simulink model "Angular_Input_Sliding_Mode_2"  (R2021b)
settings: Solver=VariableStepAuto  StartTime=0  StopTime=tspan(2)  RelTol=1e-8
undefined symbols (not defined in the file): Angle_max, BL_gain, K_switch, lambda_x_num, lambda_y_num, r_sim, tau_angle, Tmax, x_0
libraries: cstblocks x4
(part 1 of 2)
settings Model: Creator=domin  LastModifiedBy=domin
settings SolverCC: AlgebraicLoopSolver=TrustRegion
settings DataIOCC: SaveFormat=StructureWithTime
settings OptimizationCC: BlockReduction=off  BufferReuse=off
settings DebuggingCC: AlgebraicLoopMsg=none  UnconnectedInputMsg=none  UnconnectedOutputMsg=none  UnconnectedLineMsg=none  SFMachineParentedDataDiag=warning

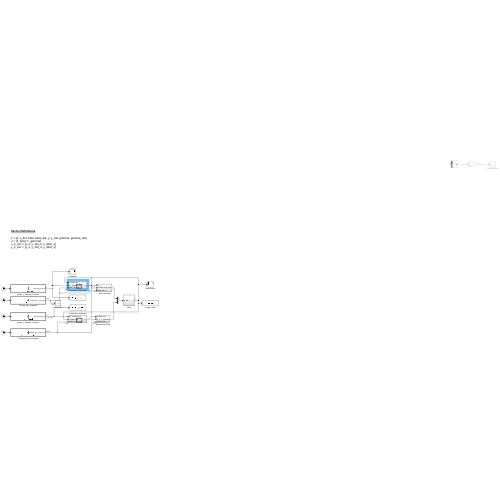
[thumbnail: Simulink's stored preview of the top-level diagram]
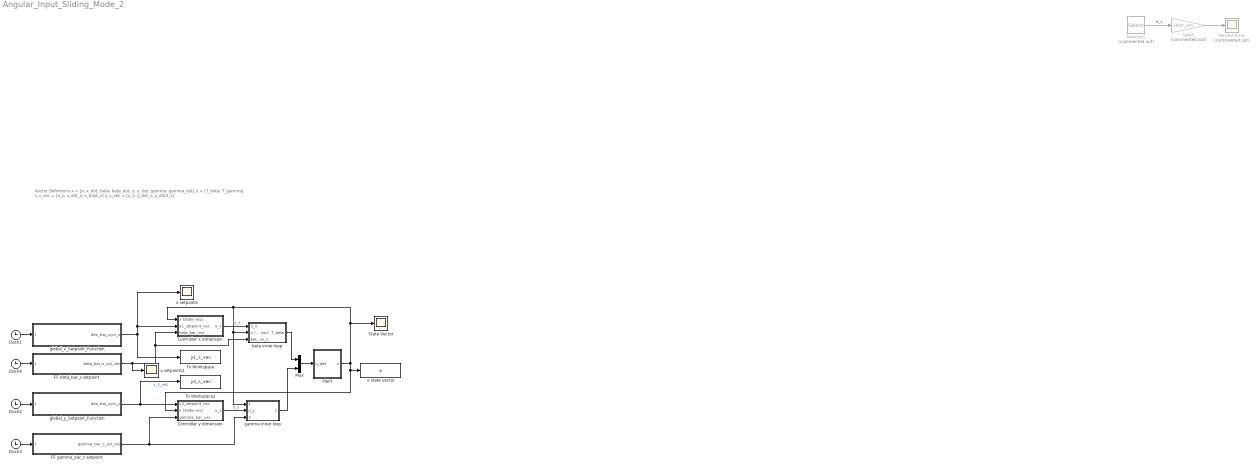
== system Angular_Input_Sliding_Mode_2 ==
  note: Vector Definitions
      |
      | x = [x; x_dot; beta; beta_dot; y; y_dot; gamma; gamma_dot]
      | u = [T_beta; T_gamma]
      | x_s_vec = [x_s; x_dot_s; x_ddot_s]
      | y_s_vec = [y_s; y_dot_s; y_ddot_s]
  Clock{1..4} (4 alike) : Clock
  Controller x dimension : Subsystem
  Controller y dimension : Subsystem
  FF beta_bar_s setpoint : MATLAB Function  TreatAsAtomicUnit=on
  FF gamma_bar_s setpoint : MATLAB Function  TreatAsAtomicUnit=on
  Gain5 : Gain  Commented=on  Gain=100/r_sim
  Mux : Mux  Inputs=2
  Percent Error : Scope  Commented=on
  Plant : Subsystem
  Selector1 : Selector  Commented=on  InputPortWidth=5  IndexOptions=Index vector (dialog)  Indices=[1]  OutputSizes=1
  State Vector : Scope
  To Workspace : ToWorkspace  VariableName=y1_s_vec  SampleTime=-1
  To Workspace2 : ToWorkspace  VariableName=y2_s_vec  SampleTime=-1
  beta inner loop : Subsystem
  gamma inner loop : Subsystem
  global_x_Setpoint_Function : MATLAB Function  TreatAsAtomicUnit=on
  global_y_Setpoint_Function : MATLAB Function  TreatAsAtomicUnit=on
  x setpoints : Scope
  x setpoints1 : Scope
  x state vector : ToWorkspace  VariableName=x  SampleTime=-1
  wires:
  Clock1/1 -> global_x_Setpoint_Function/1(t)
  Gain5/1 -> Percent Error/1
  Selector1/1 -> Gain5/1  "e_x"
  Clock2/1 -> global_y_Setpoint_Function/1(t)
  Controller x dimension/1(u_x) -> beta inner loop/1(u_x)  "u_x"
  Controller y dimension/1(u_y) -> gamma inner loop/2(u_y)  "u_y"
  global_x_Setpoint_Function/1(des_traj_sym_x) -> x setpoints/1, Controller x dimension/2(y1_setpoint_vec), To Workspace/1
  global_y_Setpoint_Function/1(des_traj_sym_y) -> To Workspace2/1, Controller y dimension/1(y2_setpoint_vec)  "y_s_vec"
  Plant/1(x) -> x state vector/1, Controller y dimension/2(x (state vec)), gamma inner loop/1(x (state vec)), beta inner loop/2(x (state vec)), Controller x dimension/1(x (state vec)), State Vector/1
  beta inner loop/1(T_beta) -> Mux/1
  Mux/1 -> Plant/1(u_des)
  gamma inner loop/1(T_gamma) -> Mux/2
  Clock3/1 -> FF gamma_bar_s setpoint/1(t)
  Clock4/1 -> FF beta_bar_s setpoint/1(t)
  FF beta_bar_s setpoint/1(beta_bar_s_sol_vec) -> x setpoints1/1, Controller x dimension/3(beta_bar_vec), beta inner loop/3(beta_bar_s)
  FF gamma_bar_s setpoint/1(gamma_bar_s_sol_vec) -> gamma inner loop/3(gamma_bar_s), Controller y dimension/3(gamma_bar_vec)

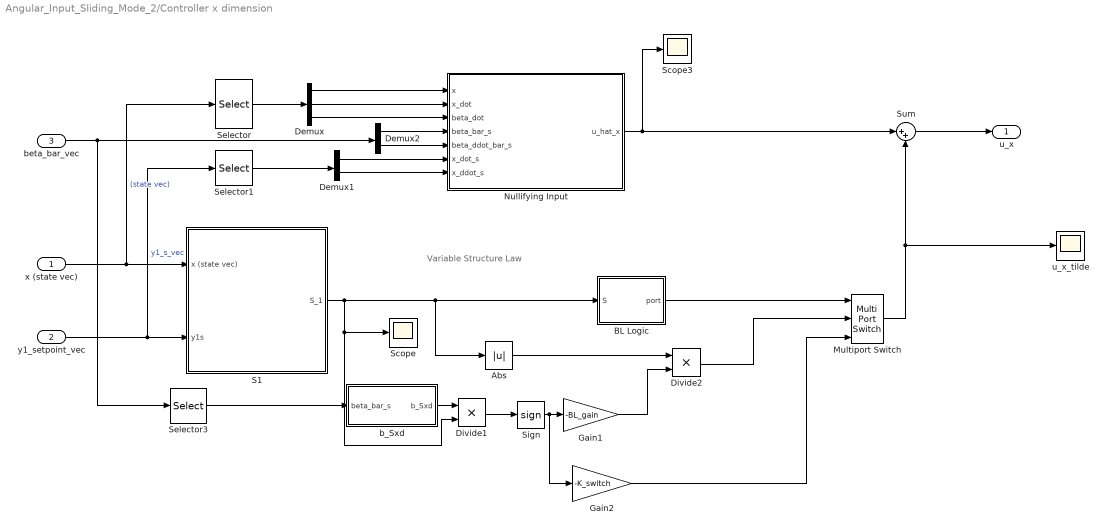
== system Angular_Input_Sliding_Mode_2/Controller x dimension ==
  note: Variable Structure Law
  x (state vec) : Inport
  y1_setpoint_vec : Inport  Port=2
  beta_bar_vec : Inport  Port=3
  Abs : Abs
  BL Logic : MATLAB Function  TreatAsAtomicUnit=on
  Demux : Demux  Outputs=3
  Demux1 : Demux  Outputs=2
  Demux2 : Demux  Outputs=2
  Divide1 : Product  Inputs=**
  Divide2 : Product  Inputs=**
  Gain1 : Gain  Gain=-BL_gain
  Gain2 : Gain  Gain=-K_switch
  Multiport Switch : MultiPortSwitch  Inputs=2
  Nullifying Input : MATLAB Function  TreatAsAtomicUnit=on
  S1 : Subsystem
  Scope : Scope
  Scope3 : Scope
  Selector : Selector  InputPortWidth=8  IndexOptions=Index vector (dialog)  Indices=[1 2 4]  OutputSizes=1
  Selector1 : Selector  InputPortWidth=3  IndexOptions=Index vector (dialog)  Indices=[2 3]  OutputSizes=1
  Selector3 : Selector  InputPortWidth=2  IndexOptions=Index vector (dialog)  Indices=[1]  OutputSizes=1
  Sign : Signum
  Sum : Sum  Inputs=|++
  b_Sxd : MATLAB Function  TreatAsAtomicUnit=on
  u_x_tilde : Scope
  u_x : Outport
  wires:
  Sum/1 -> u_x/1
  x (state vec)/1 -> S1/1(x (state vec)), Selector/1  "(state vec)"
  y1_setpoint_vec/1 -> Selector1/1, S1/2(y1s)  "y1_s_vec"
  Selector/1 -> Demux/1
  Demux/2 -> Nullifying Input/2(x_dot)
  Selector1/1 -> Demux1/1
  Demux1/1 -> Nullifying Input/6(x_dot_s)
  Demux1/2 -> Nullifying Input/7(x_ddot_s)
  Nullifying Input/1(u_hat_x) -> Scope3/1, Sum/1
  b_Sxd/1(b_Sxd) -> Divide1/1
  Divide2/1 -> Multiport Switch/2
  S1/1(S_1) -> Divide1/2, Scope/1, Abs/1, BL Logic/1(S)
  Demux/1 -> Nullifying Input/1(x)
  Gain1/1 -> Divide2/2
  BL Logic/1(port) -> Multiport Switch/1
  Multiport Switch/1 -> Sum/2, u_x_tilde/1
  Sign/1 -> Gain2/1, Gain1/1
  Divide1/1 -> Sign/1
  Gain2/1 -> Multiport Switch/3
  Abs/1 -> Divide2/1
  Demux/3 -> Nullifying Input/3(beta_dot)
  Demux2/1 -> Nullifying Input/4(beta_bar_s)
  Demux2/2 -> Nullifying Input/5(beta_ddot_bar_s)
  beta_bar_vec/1 -> Demux2/1, Selector3/1
  Selector3/1 -> b_Sxd/1(beta_bar_s)

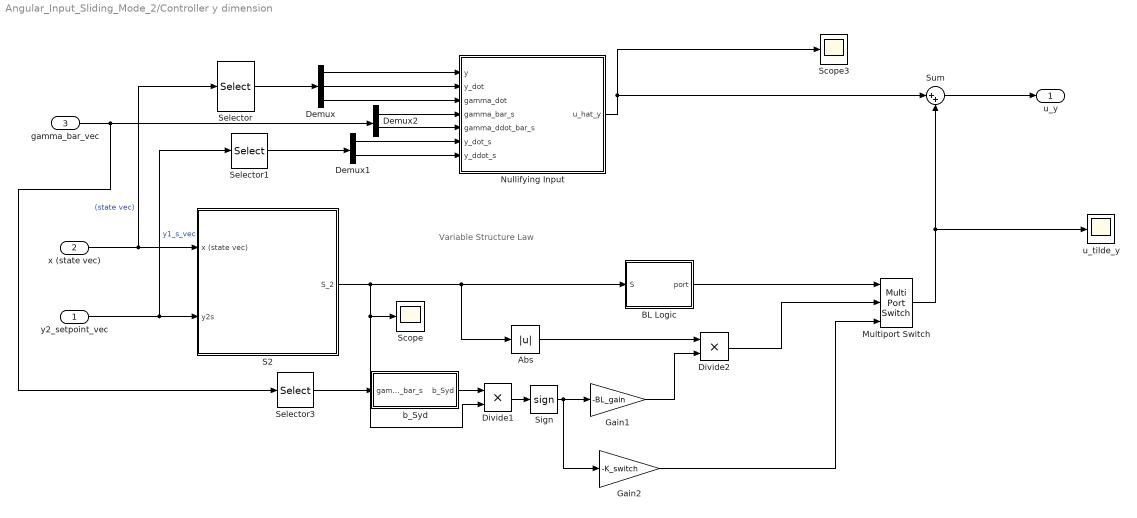
== system Angular_Input_Sliding_Mode_2/Controller y dimension ==
  note: Variable Structure Law
  y2_setpoint_vec : Inport
  x (state vec) : Inport  Port=2
  gamma_bar_vec : Inport  Port=3
  Abs : Abs
  BL Logic : MATLAB Function  TreatAsAtomicUnit=on
  Demux : Demux  Outputs=3
  Demux1 : Demux  Outputs=2
  Demux2 : Demux  Outputs=2
  Divide1 : Product  Inputs=**
  Divide2 : Product  Inputs=**
  Gain1 : Gain  Gain=-BL_gain
  Gain2 : Gain  Gain=-K_switch
  Multiport Switch : MultiPortSwitch  Inputs=2
  Nullifying Input : MATLAB Function  TreatAsAtomicUnit=on
  S2 : Subsystem
  Scope : Scope
  Scope3 : Scope
  Selector : Selector  InputPortWidth=8  IndexOptions=Index vector (dialog)  Indices=[5 6 8]  OutputSizes=1
  Selector1 : Selector  InputPortWidth=3  IndexOptions=Index vector (dialog)  Indices=[2 3]  OutputSizes=1
  Selector3 : Selector  InputPortWidth=2  IndexOptions=Index vector (dialog)  Indices=[1]  OutputSizes=1
  Sign : Signum
  Sum : Sum  Inputs=|++
  b_Syd : MATLAB Function  TreatAsAtomicUnit=on
  u_tilde_y : Scope
  u_y : Outport
  wires:
  Sum/1 -> u_y/1
  Gain1/1 -> Divide2/2
  Abs/1 -> Divide2/1
  Gain2/1 -> Multiport Switch/3
  Multiport Switch/1 -> Sum/2, u_tilde_y/1
  BL Logic/1(port) -> Multiport Switch/1
  Sign/1 -> Gain1/1, Gain2/1
  b_Syd/1(b_Syd) -> Divide1/1
  Divide2/1 -> Multiport Switch/2
  S2/1(S_2) -> Abs/1, BL Logic/1(S), Divide1/2, Scope/1
  Divide1/1 -> Sign/1
  Demux/3 -> Nullifying Input/3(gamma_dot)
  Demux/1 -> Nullifying Input/1(y)
  Nullifying Input/1(u_hat_y) -> Scope3/1, Sum/1
  Selector/1 -> Demux/1
  Demux/2 -> Nullifying Input/2(y_dot)
  x (state vec)/1 -> Selector/1, S2/1(x (state vec))  "(state vec)"
  y2_setpoint_vec/1 -> Selector1/1, S2/2(y2s)  "y1_s_vec"
  Demux1/2 -> Nullifying Input/7(y_ddot_s)
  Demux1/1 -> Nullifying Input/6(y_dot_s)
  Selector1/1 -> Demux1/1
  Selector3/1 -> b_Syd/1(gamma_bar_s)
  Demux2/1 -> Nullifying Input/4(gamma_bar_s)
  Demux2/2 -> Nullifying Input/5(gamma_ddot_bar_s)
  gamma_bar_vec/1 -> Demux2/1, Selector3/1

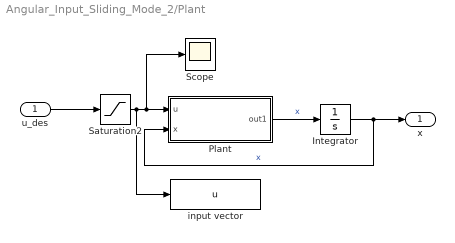
== system Angular_Input_Sliding_Mode_2/Plant ==
  u_des : Inport
  Integrator : Integrator  InitialCondition=x_0
  Plant : Subsystem
  Saturation2 : Saturate  UpperLimit=Tmax  LowerLimit=-Tmax  ZeroCross=off
  Scope : Scope
  input vector : ToWorkspace  VariableName=u  SampleTime=-1
  x : Outport
  wires:
  Saturation2/1 -> Scope/1, Plant/1(u), input vector/1
  Integrator/1 -> x/1, Plant/2(x)  "x"
  Plant/1(out1) -> Integrator/1  "x"
  u_des/1 -> Saturation2/1

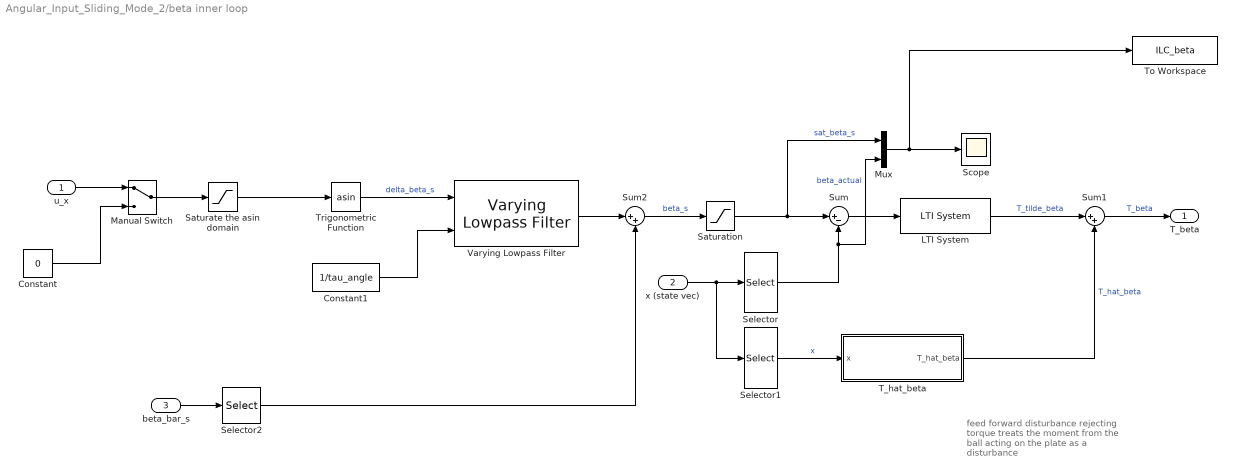
== system Angular_Input_Sliding_Mode_2/beta inner loop ==
  note: feed forward disturbance rejecting torque treats the moment from the ball acting on the plate as a disturbance
  u_x : Inport
  x (state vec) : Inport  Port=2
  beta_bar_s : Inport  Port=3
  Constant : Constant  Value=0
  Constant1 : Constant  Value=1/tau_angle
  LTI System : cstblocks/LTI System  sys=C_beta  IC=[]
  Manual Switch : ManualSwitch
  Mux : Mux  Inputs=2
  Saturate the asin domain : Saturate  UpperLimit=1  LowerLimit=-1
  Saturation : Saturate  UpperLimit=Angle_max  LowerLimit=-Angle_max
  Scope : Scope
  Selector : Selector  InputPortWidth=8  IndexOptions=Index vector (dialog)  Indices=[3]  OutputSizes=1
  Selector1 : Selector  InputPortWidth=8  IndexOptions=Index vector (dialog)  Indices=[1]  OutputSizes=1
  Selector2 : Selector  InputPortWidth=2  IndexOptions=Index vector (dialog)  Indices=[1 ]  OutputSizes=1
  Sum : Sum  Inputs=|+-
  Sum1 : Sum  Inputs=|++
  Sum2 : Sum  Inputs=|++
  T_hat_beta : MATLAB Function  TreatAsAtomicUnit=on
  To Workspace : ToWorkspace  VariableName=ILC_beta  SampleTime=-1
  Trigonometric Function : Trigonometry  Operator=asin
  Varying Lowpass Filter : cstblocks/Linear Parameter Varying/Varying Lowpass Filter  N=1
  T_beta : Outport
  wires:
  u_x/1 -> Manual Switch/1
  Trigonometric Function/1 -> Varying Lowpass Filter/1  "delta_beta_s"
  x (state vec)/1 -> Selector1/1, Selector/1
  Selector/1 -> Mux/2, Sum/2  "beta_actual"
  Sum/1 -> LTI System/1
  Saturate the asin domain/1 -> Trigonometric Function/1
  LTI System/1 -> Sum1/1  "T_tilde_beta"
  T_hat_beta/1(T_hat_beta) -> Sum1/2  "T_hat_beta"
  Sum1/1 -> T_beta/1  "T_beta"
  Selector1/1 -> T_hat_beta/1(x)  "x"
  Constant/1 -> Manual Switch/2
  Manual Switch/1 -> Saturate the asin domain/1
  Constant1/1 -> Varying Lowpass Filter/2
  Varying Lowpass Filter/1 -> Sum2/1
  Mux/1 -> To Workspace/1, Scope/1
  Saturation/1 -> Mux/1, Sum/1  "sat_beta_s"
  beta_bar_s/1 -> Selector2/1
  Selector2/1 -> Sum2/2
  Sum2/1 -> Saturation/1  "beta_s"

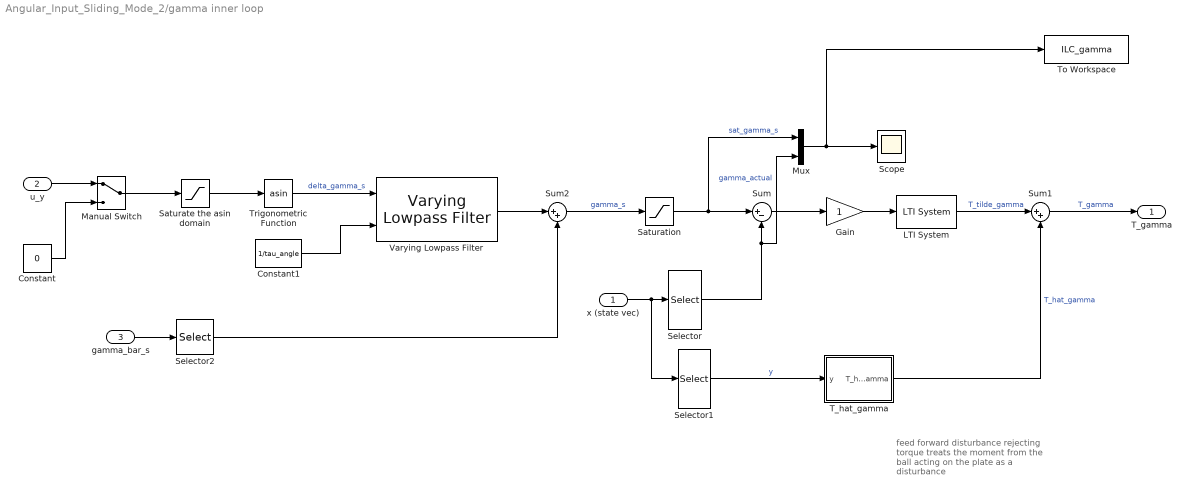
== system Angular_Input_Sliding_Mode_2/gamma inner loop ==
  note: feed forward disturbance rejecting torque treats the moment from the ball acting on the plate as a disturbance
  x (state vec) : Inport
  u_y : Inport  Port=2
  gamma_bar_s : Inport  Port=3
  Constant : Constant  Value=0
  Constant1 : Constant  Value=1/tau_angle
  Gain : Gain
  LTI System : cstblocks/LTI System  sys=C_gamma  IC=[]
  Manual Switch : ManualSwitch
  Mux : Mux  Inputs=2
  Saturate the asin domain : Saturate  UpperLimit=1  LowerLimit=-1
  Saturation : Saturate  UpperLimit=Angle_max  LowerLimit=-Angle_max
  Scope : Scope
  Selector : Selector  InputPortWidth=8  IndexOptions=Index vector (dialog)  Indices=[7]  OutputSizes=1
  Selector1 : Selector  InputPortWidth=8  IndexOptions=Index vector (dialog)  Indices=[5]  OutputSizes=1
  Selector2 : Selector  InputPortWidth=2  IndexOptions=Index vector (dialog)  Indices=[1 ]  OutputSizes=1
  Sum : Sum  Inputs=|+-
  Sum1 : Sum  Inputs=|++
  Sum2 : Sum  Inputs=|++
  T_hat_gamma : MATLAB Function  TreatAsAtomicUnit=on
  To Workspace : ToWorkspace  VariableName=ILC_gamma  SampleTime=-1
  Trigonometric Function : Trigonometry  Operator=asin
  Varying Lowpass Filter : cstblocks/Linear Parameter Varying/Varying Lowpass Filter  N=1
  T_gamma : Outport
  wires:
  LTI System/1 -> Sum1/1  "T_tilde_gamma"
  Sum/1 -> Gain/1
  Selector/1 -> Mux/2, Sum/2  "gamma_actual"
  Trigonometric Function/1 -> Varying Lowpass Filter/1  "delta_gamma_s"
  Saturation/1 -> Mux/1, Sum/1  "sat_gamma_s"
  Saturate the asin domain/1 -> Trigonometric Function/1
  T_hat_gamma/1(T_hat_gamma) -> Sum1/2  "T_hat_gamma"
  x (state vec)/1 -> Selector1/1, Selector/1
  Selector1/1 -> T_hat_gamma/1(y)  "y"
  Sum1/1 -> T_gamma/1  "T_gamma"
  u_y/1 -> Manual Switch/1
  Constant/1 -> Manual Switch/2
  Manual Switch/1 -> Saturate the asin domain/1
  Gain/1 -> LTI System/1
  Constant1/1 -> Varying Lowpass Filter/2
  Varying Lowpass Filter/1 -> Sum2/1
  Mux/1 -> To Workspace/1, Scope/1
  gamma_bar_s/1 -> Selector2/1
  Sum2/1 -> Saturation/1  "gamma_s"
  Selector2/1 -> Sum2/2

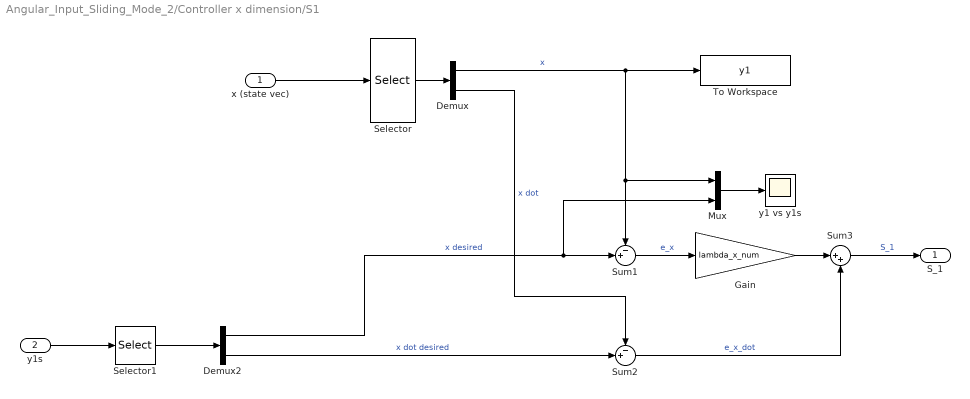
== system Angular_Input_Sliding_Mode_2/Controller x dimension/S1 ==
  x (state vec) : Inport
  y1s : Inport  Port=2
  Demux : Demux  Outputs=2
  Demux2 : Demux  Outputs=2
  Gain : Gain  Gain=lambda_x_num
  Mux : Mux  Inputs=2
  Selector : Selector  InputPortWidth=8  IndexOptions=Index vector (dialog)  Indices=[1 2]  OutputSizes=1
  Selector1 : Selector  InputPortWidth=3  IndexOptions=Index vector (dialog)  Indices=[1 2]  OutputSizes=1
  Sum1 : Sum  Inputs=-+|
  Sum2 : Sum  Inputs=-+|
  Sum3 : Sum  Inputs=|++
  To Workspace : ToWorkspace  VariableName=y1  SampleTime=-1
  y1 vs y1s : Scope
  S_1 : Outport
  wires:
  Demux/1 -> Sum1/1, Mux/1, To Workspace/1  "x"
  Demux2/2 -> Sum2/2  "x dot desired"
  Sum3/1 -> S_1/1  "S_1"
  y1s/1 -> Selector1/1
  Mux/1 -> y1 vs y1s/1
  Selector1/1 -> Demux2/1
  Selector/1 -> Demux/1
  Sum2/1 -> Sum3/2  "e_x_dot"
  Demux/2 -> Sum2/1  "x dot"
  x (state vec)/1 -> Selector/1
  Demux2/1 -> Mux/2, Sum1/2  "x desired"
  Gain/1 -> Sum3/1
  Sum1/1 -> Gain/1  "e_x"

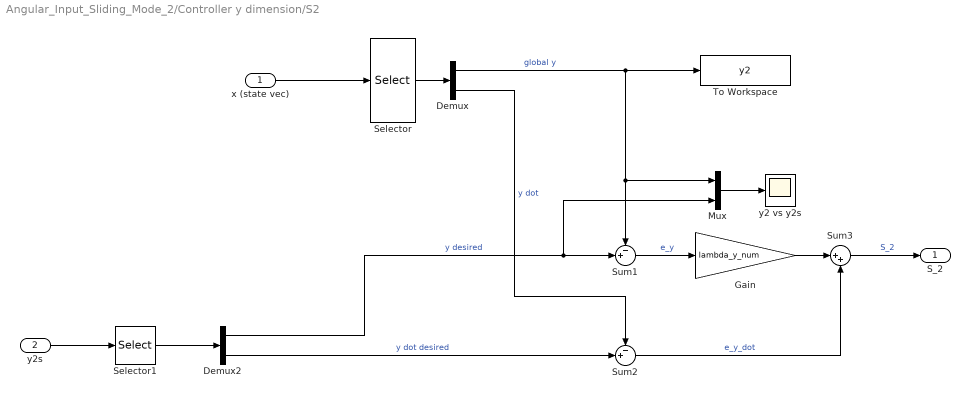
== system Angular_Input_Sliding_Mode_2/Controller y dimension/S2 ==
  x (state vec) : Inport
  y2s : Inport  Port=2
  Demux : Demux  Outputs=2
  Demux2 : Demux  Outputs=2
  Gain : Gain  Gain=lambda_y_num
  Mux : Mux  Inputs=2
  Selector : Selector  InputPortWidth=8  IndexOptions=Index vector (dialog)  Indices=[5 6]  OutputSizes=1
  Selector1 : Selector  InputPortWidth=3  IndexOptions=Index vector (dialog)  Indices=[1 2]  OutputSizes=1
  Sum1 : Sum  Inputs=-+|
  Sum2 : Sum  Inputs=-+|
  Sum3 : Sum  Inputs=|++
  To Workspace : ToWorkspace  VariableName=y2  SampleTime=-1
  y2 vs y2s : Scope
  S_2 : Outport
  wires:
  Sum3/1 -> S_2/1  "S_2"
  Sum1/1 -> Gain/1  "e_y"
  Sum2/1 -> Sum3/2  "e_y_dot"
  x (state vec)/1 -> Selector/1
  Gain/1 -> Sum3/1
  Demux/1 -> Sum1/1, Mux/1, To Workspace/1  "global y"
  Demux2/1 -> Mux/2, Sum1/2  "y desired"
  Demux2/2 -> Sum2/2  "y dot desired"
  y2s/1 -> Selector1/1
  Demux/2 -> Sum2/1  "y dot"
  Selector1/1 -> Demux2/1
  Mux/1 -> y2 vs y2s/1
  Selector/1 -> Demux/1

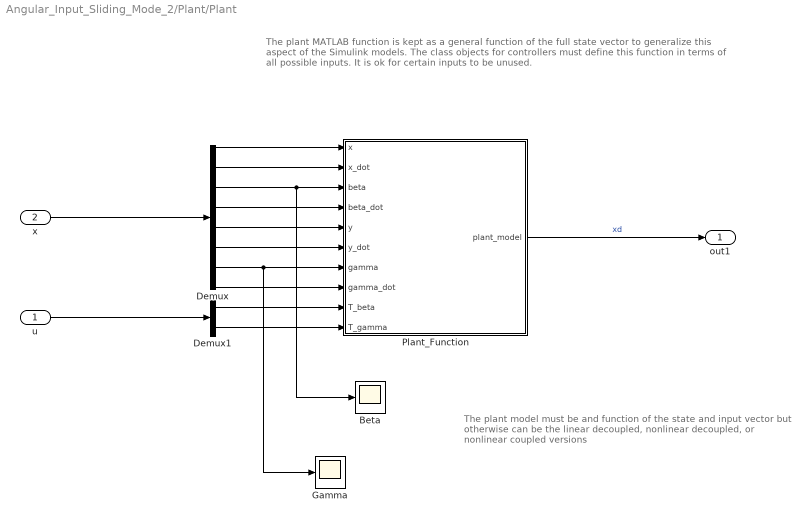
== system Angular_Input_Sliding_Mode_2/Plant/Plant ==
  note: The plant MATLAB function is kept as a general function of the full state vector
      | to generalize this aspect of the Simulink models. The class objects for controllers must define this function in terms of all possible inputs. It is ok for certain inputs to be unused.
  note: The plant model must be and function of the state and input vector
      |  but otherwise can be the linear decoupled, nonlinear decoupled,
      | or nonlinear coupled versions
  u : Inport
  x : Inport  Port=2
  Beta : Scope
  Demux : Demux  Outputs=8
  Demux1 : Demux  Outputs=2
  Gamma : Scope
  Plant_Function : MATLAB Function  TreatAsAtomicUnit=on
  out1 : Outport
  wires:
  Demux1/1 -> Plant_Function/9(T_beta)
  Demux1/2 -> Plant_Function/10(T_gamma)
  Demux/5 -> Plant_Function/5(y)
  Demux/8 -> Plant_Function/8(gamma_dot)
  Demux/1 -> Plant_Function/1(x)
  Demux/3 -> Beta/1, Plant_Function/3(beta)
  Demux/4 -> Plant_Function/4(beta_dot)
  Demux/2 -> Plant_Function/2(x_dot)
  Demux/6 -> Plant_Function/6(y_dot)
  x/1 -> Demux/1
  Plant_Function/1(plant_model) -> out1/1  "xd"
  u/1 -> Demux1/1
  Demux/7 -> Gamma/1, Plant_Function/7(gamma)

== matlab function Angular_Input_Sliding_Mode_2/FF gamma_bar_s setpoint ==
  data: t input; gamma_bar_s_sol_vec output
function gamma_bar_s_sol_vec = gamma_bar_s_vec(t)
%#codegen

%    This function was generated by the Symbolic Math Toolbox version 9.0.
%    22-Feb-2022 16:55:39

t2 = t.*pi;
t3 = pi.^2;
t4 = pi.^3;
t7 = t./2.0;
t21 = 5.151844329946315e+2;
t5 = cos(t2);
t6 = sin(t2);
t8 = t2./3.0;
t11 = -t7;
t14 = t3./9.0;
t26 = t3+6.294917864476386e+1;
t32 = t21.*(1.5e+1./9.74e+2);
t34 = t.*t21.*(-1.5e+1./9.74e+2);
t43 = t21.*3.286251181360353e-7;
t9 = t5.*pi;
t10 = t6.*pi;
t12 = cos(t8);
t13 = sin(t8);
t17 = t3.*t5;
t18 = t4.*t5;
t19 = t3.*t6;
t20 = t4.*t6;
t31 = 1.0./t26;
t33 = t.*t32;
t35 = t14+6.294917864476386e+1;
t37 = exp(t34);
t38 = t32+1.0./2.0;
t39 = t6.*t32;
t40 = t32-1.0./2.0;
t41 = t6.*t21.*(-1.5e+1./9.74e+2);
t57 = t11+t34;
t92 = t43+2.686510340762089e-3;
t96 = t43-2.686510340762089e-3;
t15 = -t9;
t16 = -t10;
t22 = (t12.*pi)./3.0;
t23 = (t13.*pi)./3.0;
t27 = t12.*t14;
t28 = (t4.*t12)./2.7e+1;
t29 = t13.*t14;
t30 = (t4.*t13)./2.7e+1;
t36 = exp(t33);
t42 = t9.*t32;
t44 = 1.0./t35;
t45 = t38.^2;
t46 = t9.*t21.*(-1.5e+1./9.74e+2);
t47 = t19.*t32;
t48 = t13.*t32;
t49 = t40.^2;
t50 = t12.*t21.*pi.*(5.0./9.74e+2);
t51 = t13.*t21.*(-1.5e+1./9.74e+2);
t52 = t11+t33;
t54 = t5.*t38;
t55 = t3.*t13.*t21.*1.711156741957563e-3;
t56 = t6.*t38;
t59 = t5.*t40;
t60 = t6.*t40;
t61 = t9.*t38;
t62 = t10.*t38;
t64 = exp(t57);
t65 = t9.*t40;
t66 = t10.*t40;
t68 = t9+t39;
t69 = t12.*t38;
t70 = t13.*t38;
t72 = t19.*t38;
t73 = t9+t41;
t74 = t12.*t40;
t75 = t13.*t40;
t77 = t19.*t40;
t24 = -t22;
t25 = -t23;
t53 = -t50;
t58 = exp(t52);
t63 = t3+t45;
t67 = t3+t49;
t71 = t15.*t38;
t76 = t16.*t40;
t79 = t19+t42;
t81 = t19+t46;
t82 = -t77;
t83 = t14+t45;
t84 = t22.*t38;
t85 = t23.*t38;
t86 = t9+t56;
t87 = t14+t49;
t88 = t22.*t40;
t89 = t69.*pi.*(-1.0./3.0);
t90 = t23.*t40;
t91 = t10+t59;
t94 = t75.*pi.*(-1.0./3.0);
t95 = t16+t54;
t98 = t17+t62;
t99 = t15+t60;
t100 = t29.*t38;
t101 = t19+t65;
t102 = t29.*t40;
t103 = t22+t48;
t105 = t18+t72;
t106 = t3.*t75.*(-1.0./9.0);
t107 = t22+t51;
t109 = t29+t50;
t112 = t22+t70;
t113 = t23+t74;
t123 = t64.*t96;
t124 = t3.*t21.*t31.*t37.*t68.*1.648361999133433e-4;
t125 = t3.*t21.*t31.*t36.*t73.*1.648361999133433e-4;
t78 = 1.0./t63;
t80 = 1.0./t67;
t93 = 1.0./t83;
t97 = 1.0./t87;
t104 = t19+t71;
t108 = t17+t76;
t110 = t29+t53;
t111 = t18+t82;
t114 = t25+t69;
t115 = t24+t75;
t116 = t27+t85;
t117 = t29+t88;
t118 = t29+t89;
t119 = t27+t94;
t120 = t28+t100;
t121 = t28+t106;
t122 = t58.*t92;
t126 = -t124;
t127 = -t125;
t128 = t3.*t21.*t37.*t44.*t103.*1.831513332370481e-5;
t129 = t3.*t21.*t36.*t44.*t107.*1.831513332370481e-5;
t130 = t21.*t64.*t78.*t86.*4.120904997833581e-5;
t132 = t21.*t58.*t80.*t91.*pi.*1.648361999133433e-4;
t134 = t21.*t64.*t78.*pi.*(t10-t54).*(-1.648361999133433e-4);
t135 = t3.*t21.*t64.*t78.*t86.*1.648361999133433e-4;
t136 = t21.*t58.*t80.*(t9-t60).*(-4.120904997833581e-5);
t137 = t3.*t21.*t58.*t80.*(t9-t60).*(-1.648361999133433e-4);
t138 = t3.*t21.*t58.*t80.*(t9-t60).*1.648361999133433e-4;
t139 = t21.*t64.*t93.*t112.*4.120904997833581e-5;
t140 = t21.*t58.*t97.*(t22-t75).*(-4.120904997833581e-5);
t141 = t21.*t64.*t93.*pi.*(t23-t69).*(-5.494539997111442e-5);
t142 = t21.*t58.*t97.*t113.*pi.*5.494539997111442e-5;
t143 = t3.*t21.*t64.*t93.*t112.*1.831513332370481e-5;
t144 = t21.*t58.*t97.*(t22-t75).*4.120904997833581e-5;
t145 = t21.*t64.*t93.*pi.*(t23-t69).*5.494539997111442e-5;
t147 = t3.*t21.*t58.*t97.*(t22-t75).*(-1.831513332370481e-5);
t131 = -t130;
t133 = -t132;
t146 = -t143;
t148 = t123+t126+t128+t131+t134+t135+t139+t145+t146;
t149 = t122+t127+t129+t133+t136+t138+t142+t144+t147;
et1 = t45.*t123+t45.*t134+t45.*t135+t45.*t139+t45.*t145-t3.*t31.*t37.*t81.*1.347535934291581+t3.*t37.*t44.*t110.*1.497262149212868e-1+t21.*t64.*t78.*t105.*4.120904997833581e-5-t21.*t64.*t93.*t120.*4.120904997833581e-5+t21.*t64.*t78.*pi.*(t20-t17.*t38).*1.648361999133433e-4-t21.*t64.*t93.*pi.*(t30-(t3.*t69)./9.0).*5.494539997111442e-5+t3.*t21.*t31.*t37.*(t18+t47).*1.648361999133433e-4-t3.*t21.*t37.*t44.*(t28+t55).*1.831513332370481e-5-t3.*t21.*t31.*t37.*t68.*1.037630339546905e-2+t3.*t21.*t37.*t44.*t103.*1.152922599496562e-3;
et2 = t3.*t21.*t64.*t78.*t105.*(-1.648361999133433e-4)-t21.*t45.*t64.*t78.*t86.*4.120904997833581e-5+t3.*t21.*t64.*t93.*t120.*1.831513332370481e-5-t21.*t38.*t64.*t78.*t104.*8.241809995667163e-5+t21.*t38.*t64.*t93.*t118.*8.241809995667163e-5+t3.*t21.*t38.*t64.*t78.*t104.*3.296723998266865e-4-t3.*t21.*t38.*t64.*t93.*t118.*3.663026664740961e-5-t3.*t21.*t45.*t64.*t93.*t112.*1.831513332370481e-5+t21.*t38.*t64.*t78.*t98.*pi.*3.296723998266865e-4-t21.*t38.*t64.*t93.*t116.*pi.*1.098907999422288e-4;
et3 = t49.*t122+t49.*t136+t49.*t138+t49.*t142+t49.*t144+t49.*t147+t3.*t31.*t36.*t79.*1.347535934291581-t3.*t36.*t44.*t109.*1.497262149212868e-1+t21.*t58.*t80.*t111.*4.120904997833581e-5-t21.*t58.*t97.*t121.*4.120904997833581e-5+t21.*t58.*t80.*pi.*(t20+t17.*t40).*1.648361999133433e-4-t21.*t58.*t97.*pi.*(t30+t27.*t40).*5.494539997111442e-5+t3.*t21.*t31.*t36.*(t18-t19.*t21.*(1.5e+1./9.74e+2)).*1.648361999133433e-4-t3.*t21.*t31.*t36.*t73.*1.037630339546905e-2+t3.*t21.*t36.*t44.*t107.*1.152922599496562e-3-t3.*t21.*t58.*t80.*t111.*1.648361999133433e-4;
et4 = t3.*t21.*t58.*t97.*t121.*1.831513332370481e-5+t21.*t40.*t58.*t80.*t101.*8.241809995667163e-5-t21.*t40.*t58.*t97.*t117.*8.241809995667163e-5-t3.*t21.*t36.*t44.*(t28-t55).*1.831513332370481e-5-t3.*t21.*t40.*t58.*t80.*t101.*3.296723998266865e-4+t3.*t21.*t40.*t58.*t97.*t117.*3.663026664740961e-5-t21.*t49.*t58.*t80.*t91.*pi.*1.648361999133433e-4-t21.*t40.*t58.*t80.*t108.*pi.*3.296723998266865e-4+t21.*t40.*t58.*t97.*t119.*pi.*1.098907999422288e-4;
et5 = t38.*t123+t38.*t134+t38.*t135+t38.*t139+t38.*t145-t3.*t31.*t37.*t68.*6.737679671457906e-1+t3.*t37.*t44.*t103.*7.486310746064339e-2-t21.*t64.*t78.*t104.*4.120904997833581e-5+t21.*t64.*t93.*t118.*4.120904997833581e-5+t21.*t64.*t78.*t98.*pi.*1.648361999133433e-4-t21.*t64.*t93.*t116.*pi.*5.494539997111442e-5-t3.*t21.*t31.*t37.*t81.*1.648361999133433e-4+t3.*t21.*t37.*t44.*t110.*1.831513332370481e-5+t3.*t21.*t64.*t78.*t104.*1.648361999133433e-4-t21.*t38.*t64.*t78.*t86.*4.120904997833581e-5-t3.*t21.*t64.*t93.*t118.*1.831513332370481e-5;
et6 = t3.*t21.*t38.*t64.*t93.*t112.*(-1.831513332370481e-5);
et7 = t21.*t37.*(t40.*t122+t40.*t136+t40.*t138+t40.*t142+t40.*t144+t40.*t147-t3.*t31.*t36.*t73.*6.737679671457906e-1+t3.*t36.*t44.*t107.*7.486310746064339e-2+t21.*t58.*t80.*t101.*4.120904997833581e-5-t21.*t58.*t97.*t117.*4.120904997833581e-5-t21.*t58.*t80.*t108.*pi.*1.648361999133433e-4+t21.*t58.*t97.*t119.*pi.*5.494539997111442e-5+t3.*t21.*t31.*t36.*t79.*1.648361999133433e-4-t3.*t21.*t36.*t44.*t109.*1.831513332370481e-5-t3.*t21.*t58.*t80.*t101.*1.648361999133433e-4+t3.*t21.*t58.*t97.*t117.*1.831513332370481e-5-t21.*t40.*t58.*t80.*t91.*pi.*1.648361999133433e-4);
et8 = 1.5e+1./4.87e+2;
gamma_bar_s_sol_vec = [t36.*t148-t37.*t149;t36.*(et1+et2)+t36.*t148.*6.294917864476386e+1-t37.*t149.*6.294917864476386e+1-t37.*(et3+et4)-t21.*t36.*(et5+et6).*(1.5e+1./4.87e+2)+et7.*et8];

== matlab function Angular_Input_Sliding_Mode_2/Controller x dimension/BL Logic ==
  data: S input; port output; S_BL_value parameter
function port = fcn(S,S_BL_value)

if abs(S) <= S_BL_value

    port = 1; %If we are in the boundary layer, use the boundary layer proportional law

else 
    port = 2; %Outside, use the signum law
end

== matlab function Angular_Input_Sliding_Mode_2/Controller x dimension/b_Sxd ==
  data: beta_bar_s input; b_Sxd output
function b_Sxd = b_Sxd(beta_bar_s)
%#codegen

%    This function was generated by the Symbolic Math Toolbox version 9.0.
%    22-Feb-2022 16:55:40

b_Sxd = [cos(beta_bar_s).*(-9.81e+2./1.4e+2)];

== matlab function Angular_Input_Sliding_Mode_2/Controller y dimension/b_Syd ==
  data: gamma_bar_s input; b_Syd output
function b_Syd = b_Syd(gamma_bar_s)
%#codegen

%    This function was generated by the Symbolic Math Toolbox version 9.0.
%    22-Feb-2022 16:55:40

b_Syd = [cos(gamma_bar_s).*(9.81e+2./1.4e+2)];
